simulink model "Kfilter"  (R2017b)
settings: Solver=FixedStepAuto  StartTime=0.0  StopTime=50  FixedStep=interval  RelTol=1e-3
undefined symbols (not defined in the file or in its folder): interval, KfilterQ, KfilterR
settings Model: Creator=schapman  LastModifiedBy=schapman

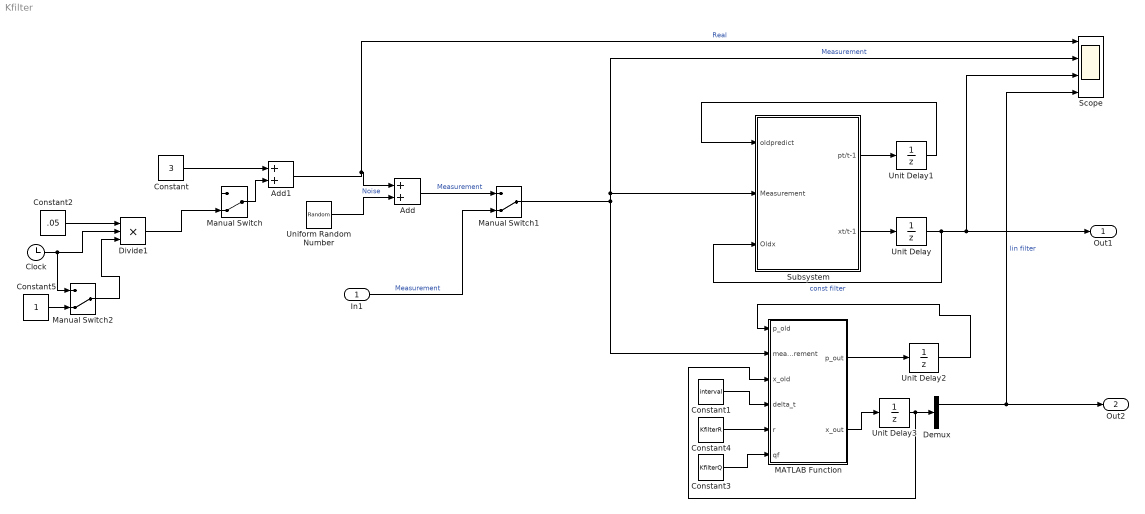
== system Kfilter ==
  In1 : Inport
  Add : Sum
  Add1 : Sum
  Clock : Clock
  Constant : Constant  Value=3
  Constant1 : Constant  Value=interval
  Constant2 : Constant  Value=.05
  Constant3 : Constant  Value=KfilterQ
  Constant4 : Constant  Value=KfilterR
  Constant5 : Constant
  Demux : Demux  Outputs=2
  Divide1 : Product  Inputs=***
  MATLAB Function : MATLAB Function  TreatAsAtomicUnit=on
  Manual Switch : ManualSwitch  CurrentSetting=0
  Manual Switch1 : ManualSwitch  CurrentSetting=0
  Manual Switch2 : ManualSwitch  CurrentSetting=0
  Scope : Scope  NumInputPorts=4
  Subsystem : Subsystem
  Uniform Random Number : UniformRandomNumber  Minimum=-.5  Maximum=.5  Seed=5  SampleTime=0.05
  Unit Delay : UnitDelay  SampleTime=-1
  Unit Delay1 : UnitDelay  InitialCondition=1000  SampleTime=-1
  Unit Delay2 : UnitDelay  InitialCondition=[1000,0;0,1000]  SampleTime=-1
  Unit Delay3 : UnitDelay  InitialCondition=[0;0]  SampleTime=-1
  Out1 : Outport
  Out2 : Outport  Port=2
  wires:
  Add1/1 -> Scope/1, Add/1  "Real"
  Uniform Random Number/1 -> Add/2  "Noise"
  Manual Switch1/1 -> MATLAB Function/2(measurement), Scope/2, Subsystem/2(Measurement)  "Measurement"
  Subsystem/2(xt/t-1) -> Unit Delay/1
  Unit Delay/1 -> Scope/3, Out1/1, Subsystem/3(Oldx)  "const filter"
  Subsystem/1(pt/t-1) -> Unit Delay1/1
  Unit Delay1/1 -> Subsystem/1(oldpredict)
  Constant1/1 -> MATLAB Function/4(delta_t)
  MATLAB Function/1(p_out) -> Unit Delay2/1
  Unit Delay2/1 -> MATLAB Function/1(p_old)
  MATLAB Function/2(x_out) -> Unit Delay3/1
  Unit Delay3/1 -> Demux/1, MATLAB Function/3(x_old)
  Demux/1 -> Out2/1, Scope/4  "lin filter"
  Constant/1 -> Add1/1
  Constant2/1 -> Divide1/1
  Clock/1 -> Manual Switch2/1, Divide1/2
  Divide1/1 -> Manual Switch/2
  Constant4/1 -> MATLAB Function/5(r)
  Constant3/1 -> MATLAB Function/6(qf)
  Manual Switch/1 -> Add1/2
  Add/1 -> Manual Switch1/1  "Measurement"
  In1/1 -> Manual Switch1/2  "Measurement"
  Constant5/1 -> Manual Switch2/2
  Manual Switch2/1 -> Divide1/3

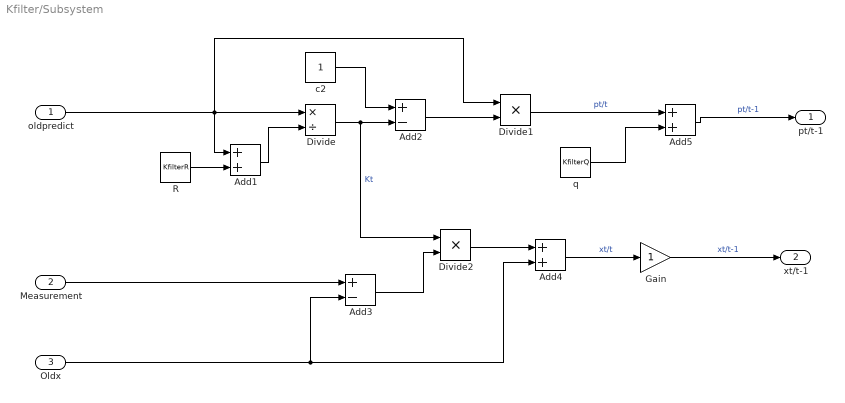
== system Kfilter/Subsystem ==
  oldpredict : Inport
  Measurement : Inport  Port=2
  Oldx : Inport  Port=3
  Add1 : Sum
  Add2 : Sum  Inputs=+-
  Add3 : Sum  Inputs=+-
  Add4 : Sum
  Add5 : Sum
  Divide : Product  Inputs=*/
  Divide1 : Product  Inputs=**
  Divide2 : Product  Inputs=**
  Gain : Gain
  R : Constant  Value=KfilterR
  c2 : Constant
  q : Constant  Value=KfilterQ
  pt/t-1 : Outport
  xt/t-1 : Outport  Port=2
  wires:
  c2/1 -> Add2/1
  R/1 -> Add1/2
  Add2/1 -> Divide1/2
  Oldx/1 -> Add3/2, Add4/2
  Add3/1 -> Divide2/2
  Divide1/1 -> Add5/1  "pt/t"
  oldpredict/1 -> Divide1/1, Add1/1, Divide/1
  Measurement/1 -> Add3/1
  Add1/1 -> Divide/2
  q/1 -> Add5/2
  Add5/1 -> pt/t-1/1  "pt/t-1"
  Divide/1 -> Divide2/1, Add2/2  "Kt"
  Add4/1 -> Gain/1  "xt/t"
  Divide2/1 -> Add4/1
  Gain/1 -> xt/t-1/1  "xt/t-1"

== matlab function Kfilter/MATLAB Function ==
  data: p_old input; p_out output; measurement input; x_old input; delta_t input; x_out output; r input; qf input
function [p_out,x_out] = fcn(p_old,measurement,x_old, delta_t,r, qf)

Q = [delta_t^3*qf/3, delta_t^2*qf/2; delta_t^2*qf/2, delta_t*qf];
F = [1, delta_t;0,1];
H = [1,0];

Kt=p_old*transpose(H)*inv(H*p_old*transpose(H)+r);
xcurrent=x_old+Kt*(measurement-H*x_old);
pcurrent=(eye(2)-Kt*H)*p_old;

p_out = F*pcurrent*transpose(F)+Q;
x_out = F*xcurrent;

end
